simulink model "updated_target_driver_2026_withVariants_MPC"  (R2024b)
settings: Solver=FixedStepDiscrete  StartTime=0.0  StopTime=running_time  FixedStep=dt_s  RelTol=1e-3
values from neighbouring files (symbols this model uses):
  A = gamma_2*gamma_3*Thrust_desired    [force2voltage.m]
  a2_lb = -0.25    [target_driver_setup_2022_Ctrl_V_2_4.m]    (also in target_driver_setup_2022_Ctrl_V_2_4_geometric.m; target_driver_setup_mpc_12msdelay.m; target_driver_setup_mpc_andWLQP.m)
  a2_openloop = -0    (= 0)    [target_driver_setup_2022_Ctrl_V_2_4.m]    (also in target_driver_setup_2022_Ctrl_V_2_4_geometric.m; target_driver_setup_mpc_12msdelay.m; target_driver_setup_mpc_andWLQP.m)
  a2_ub = 0.25    [target_driver_setup_2022_Ctrl_V_2_4.m]    (also in target_driver_setup_2022_Ctrl_V_2_4_geometric.m; target_driver_setup_mpc_12msdelay.m; target_driver_setup_mpc_andWLQP.m)
  adaptive_flag = 0    [target_driver_setup_2022_Ctrl_V_2_4.m]    (also in target_driver_setup_2022_Ctrl_V_2_4_geometric.m; target_driver_setup_mpc_12msdelay.m = 1; target_driver_setup_mpc_andWLQP.m = 1)
  adaptive_gain = [gamma_adaptive, adaptive_roll_limit, adaptive_pitch_limit, adaptive_yaw_limit, c_2_adaptive, gamma_lateral_adaptive, adaptive_x_limit, adaptive_y_limit, adaptive_z_limit, c_1_adaptive]    [target_driver_setup_2022_Ctrl_V_2_4.m]    (also in target_driver_setup_2022_Ctrl_V_2_4_geometric.m; target_driver_setup_mpc_12msdelay.m; target_driver_setup_mpc_andWLQP.m)
  adaptive_lateral_flag = 0    [target_driver_setup_2022_Ctrl_V_2_4.m]    (also in target_driver_setup_2022_Ctrl_V_2_4_geometric.m; target_driver_setup_mpc_12msdelay.m = 1; target_driver_setup_mpc_andWLQP.m = 1)
  adaptive_pitch_init = 0    [target_driver_setup_2022_Ctrl_V_2_4.m]    (also in target_driver_setup_2022_Ctrl_V_2_4_geometric.m; target_driver_setup_mpc_12msdelay.m; target_driver_setup_mpc_andWLQP.m)
  adaptive_pitch_limit = 0.1/(scale^2)    (= 1e-07)    [target_driver_setup_2022_Ctrl_V_2_4.m]    (also in target_driver_setup_2022_Ctrl_V_2_4_geometric.m = 3e-07; target_driver_setup_mpc_12msdelay.m; target_driver_setup_mpc_andWLQP.m)
  adaptive_pitch_limit_low = -adaptive_pitch_limit    (= -1e-07)    [target_driver_setup_2022_Ctrl_V_2_4.m]    (also in target_driver_setup_2022_Ctrl_V_2_4_geometric.m = -3e-07; target_driver_setup_mpc_12msdelay.m; target_driver_setup_mpc_andWLQP.m)
  adaptive_roll_init = 0    [target_driver_setup_2022_Ctrl_V_2_4.m]    (also in target_driver_setup_2022_Ctrl_V_2_4_geometric.m; target_driver_setup_mpc_12msdelay.m; target_driver_setup_mpc_andWLQP.m)
  adaptive_roll_limit = 0.3/(scale^2)    (= 3e-07)    [target_driver_setup_2022_Ctrl_V_2_4.m]    (also in target_driver_setup_2022_Ctrl_V_2_4_geometric.m; target_driver_setup_mpc_12msdelay.m; target_driver_setup_mpc_andWLQP.m)
  adaptive_roll_limit_low = -adaptive_roll_limit    (= -3e-07)    [target_driver_setup_2022_Ctrl_V_2_4.m]    (also in target_driver_setup_2022_Ctrl_V_2_4_geometric.m; target_driver_setup_mpc_12msdelay.m; target_driver_setup_mpc_andWLQP.m)
  adaptive_x_init = 0    [target_driver_setup_2022_Ctrl_V_2_4.m]    (also in target_driver_setup_2022_Ctrl_V_2_4_geometric.m; target_driver_setup_mpc_12msdelay.m; target_driver_setup_mpc_andWLQP.m)
  adaptive_x_limit = 0.15/(scale)    (= 0.00015)    [target_driver_setup_2022_Ctrl_V_2_4.m]    (also in target_driver_setup_2022_Ctrl_V_2_4_geometric.m = 7.5e-05; target_driver_setup_mpc_12msdelay.m; target_driver_setup_mpc_andWLQP.m)
  adaptive_x_limit_low = -adaptive_x_limit    (= -0.00015)    [target_driver_setup_2022_Ctrl_V_2_4.m]    (also in target_driver_setup_2022_Ctrl_V_2_4_geometric.m = -7.5e-05; target_driver_setup_mpc_12msdelay.m; target_driver_setup_mpc_andWLQP.m)
  adaptive_y_init = 0    [target_driver_setup_2022_Ctrl_V_2_4.m]    (also in target_driver_setup_2022_Ctrl_V_2_4_geometric.m; target_driver_setup_mpc_12msdelay.m; target_driver_setup_mpc_andWLQP.m)
  adaptive_y_limit = 0.15/(scale)    (= 0.00015)    [target_driver_setup_2022_Ctrl_V_2_4.m]    (also in target_driver_setup_2022_Ctrl_V_2_4_geometric.m = 7.5e-05; target_driver_setup_mpc_12msdelay.m; target_driver_setup_mpc_andWLQP.m)
  adaptive_y_limit_low = -adaptive_y_limit    (= -0.00015)    [target_driver_setup_2022_Ctrl_V_2_4.m]    (also in target_driver_setup_2022_Ctrl_V_2_4_geometric.m = -7.5e-05; target_driver_setup_mpc_12msdelay.m; target_driver_setup_mpc_andWLQP.m)
  adaptive_yaw_init = 0    [target_driver_setup_2022_Ctrl_V_2_4.m]    (also in target_driver_setup_2022_Ctrl_V_2_4_geometric.m; target_driver_setup_mpc_12msdelay.m; target_driver_setup_mpc_andWLQP.m)
  adaptive_yaw_limit = 0.035/(scale^2)    (= 3.5e-08)    [target_driver_setup_2022_Ctrl_V_2_4.m]    (also in target_driver_setup_2022_Ctrl_V_2_4_geometric.m; target_driver_setup_mpc_12msdelay.m; target_driver_setup_mpc_andWLQP.m)
  adaptive_yaw_limit_low = -adaptive_yaw_limit    (= -3.5e-08)    [target_driver_setup_2022_Ctrl_V_2_4.m]    (also in target_driver_setup_2022_Ctrl_V_2_4_geometric.m; target_driver_setup_mpc_12msdelay.m; target_driver_setup_mpc_andWLQP.m)
  adaptive_z_init = 0/scale    (= 0)    [target_driver_setup_2022_Ctrl_V_2_4.m]    (also in target_driver_setup_2022_Ctrl_V_2_4_geometric.m; target_driver_setup_mpc_12msdelay.m; target_driver_setup_mpc_andWLQP.m)
  adaptive_z_limit = 0.20/(scale)    (= 0.0002)    [target_driver_setup_2022_Ctrl_V_2_4.m]    (also in target_driver_setup_2022_Ctrl_V_2_4_geometric.m = 0.0008; target_driver_setup_mpc_12msdelay.m = 0.0008; target_driver_setup_mpc_andWLQP.m = 0.0008)
  adaptive_z_limit_low = -adaptive_z_limit/1    (= -0.0002)    [target_driver_setup_2022_Ctrl_V_2_4.m]    (also in target_driver_setup_2022_Ctrl_V_2_4_geometric.m = -0.0008; target_driver_setup_mpc_12msdelay.m = -0.0008; target_driver_setup_mpc_andWLQP.m = -0.0008)
  att_s = 500    [target_driver_setup_2022_Ctrl_V_2_4.m]    (also in target_driver_setup_2022_Ctrl_V_2_4_geometric.m; target_driver_setup_mpc_12msdelay.m; target_driver_setup_mpc_andWLQP.m)
  b_1_d_desired = [1,0,0]    [target_driver_setup_2022_Ctrl_V_2_4.m]    (also in target_driver_setup_2022_Ctrl_V_2_4_geometric.m; target_driver_setup_mpc_12msdelay.m; target_driver_setup_mpc_andWLQP.m)
  closedloop_flag = 1    [target_driver_setup_2022_Ctrl_V_2_4.m]    (also in target_driver_setup_2022_Ctrl_V_2_4_geometric.m = 0; target_driver_setup_mpc_12msdelay.m = 0; target_driver_setup_mpc_andWLQP.m = 0)
  control_gain = [k_x,k_v, k_R, k_Omega, k_z, k_vz, k_Rx]    [target_driver_setup_2022_Ctrl_V_2_4.m]    (also in target_driver_setup_2022_Ctrl_V_2_4_geometric.m = [k_x,k_v,k_R,k_Omega_pitch,k_Omega_roll,k_z,k_vz,k_Rx]; target_driver_setup_mpc_12msdelay.m = [k_x, k_v, k_R, k_Omega, k_z, k_vz, k_Rx,                  k; target_driver_setup_mpc_andWLQP.m = [k_x, k_v, k_R, k_Omega, k_z, k_vz, k_Rx,                  k)
  delay = delay-vicon_sample_cycle/2    [target_driver_setup_2022_Ctrl_V_2_4.m]    (also in target_driver_setup_2022_Ctrl_V_2_4_geometric.m; target_driver_setup_mpc_12msdelay.m; target_driver_setup_mpc_andWLQP.m)
  drv_amp = abs((vleft_p2p-vright_p2p))/2+min(vleft_p2p,vright_p2p)    [Wing_traj_to_Voltage.m]    (also in force2voltage.m; target_driver_setup_2022_Ctrl_V_2_4.m = 300; target_driver_setup_2022_Ctrl_V_2_4_geometric.m = 133; target_driver_setup_mpc_12msdelay.m = 150)
  drv_bias = max_drv_bias    (= 300)    [target_driver_setup_2022_Ctrl_V_2_4.m]    (also in target_driver_setup_2022_Ctrl_V_2_4_geometric.m = 200; target_driver_setup_mpc_12msdelay.m = 200; target_driver_setup_mpc_andWLQP.m = 200)
  drv_pitch_left = vleft_pitch    [Wing_traj_to_Voltage.m]    (also in force2voltage.m = 0; target_driver_setup_2022_Ctrl_V_2_4.m = 0; target_driver_setup_2022_Ctrl_V_2_4_geometric.m = 0; target_driver_setup_mpc_12msdelay.m = 9.05)
  drv_pitch_right = vright_pitch    [Wing_traj_to_Voltage.m]    (also in force2voltage.m = 0; target_driver_setup_2022_Ctrl_V_2_4.m = 0; target_driver_setup_2022_Ctrl_V_2_4_geometric.m = 0; target_driver_setup_mpc_12msdelay.m = 9.05)
  drv_roll = (vleft_p2p-vright_p2p)/4    [Wing_traj_to_Voltage.m]    (also in force2voltage.m; target_driver_setup_2022_Ctrl_V_2_4.m = 0; target_driver_setup_2022_Ctrl_V_2_4_geometric.m = -0.001; target_driver_setup_mpc_12msdelay.m = -0.001)
  dt_s = 1e-3    (= 0.001)    [target_driver_setup_2022_Ctrl_V_2_4.m]    (also in target_driver_setup_2022_Ctrl_V_2_4_geometric.m = 0.0002; target_driver_setup_mpc_12msdelay.m = 0.0002; target_driver_setup_mpc_andWLQP.m = 0.0002)
  f_fin = f    (= 180)    [target_driver_setup_2022_Ctrl_V_2_4.m]    (also in target_driver_setup_2022_Ctrl_V_2_4_geometric.m = 155; target_driver_setup_mpc_12msdelay.m = 155; target_driver_setup_mpc_andWLQP.m = 155)
  f_int = f    (= 180)    [target_driver_setup_2022_Ctrl_V_2_4.m]    (also in target_driver_setup_2022_Ctrl_V_2_4_geometric.m = 155; target_driver_setup_mpc_12msdelay.m = 155; target_driver_setup_mpc_andWLQP.m = 155)
  g = 9.8    [target_driver_setup_2022_Ctrl_V_2_4.m]    (also in target_driver_setup_2022_Ctrl_V_2_4_geometric.m; target_driver_setup_mpc_12msdelay.m; target_driver_setup_mpc_andWLQP.m = 9.81; test_full_attitude_mpc.m = 9.81)
  I_moment_vec = [Ixx, Iyy, Izz]    [target_driver_setup_2022_Ctrl_V_2_4.m]    (also in target_driver_setup_2022_Ctrl_V_2_4_geometric.m; target_driver_setup_mpc_12msdelay.m; target_driver_setup_mpc_andWLQP.m)
  k_tau_vec = [k_tau_roll;k_tau_pitch]    [target_driver_setup_2022_Ctrl_V_2_4_geometric.m]    (also in target_driver_setup_mpc_12msdelay.m; target_driver_setup_mpc_andWLQP.m)
  landing_flag = 0    [target_driver_setup_2022_Ctrl_V_2_4.m]    (also in target_driver_setup_2022_Ctrl_V_2_4_geometric.m; target_driver_setup_mpc_12msdelay.m; target_driver_setup_mpc_andWLQP.m)
  landing_parameter = [start_delay+T,transition_rate, rising_time, falling_time, landing_rising_time, landing_z_decrease, landing_y_decrease, landing_x_decrease]    [target_driver_setup_2022_Ctrl_V_2_4.m]    (also in target_driver_setup_2022_Ctrl_V_2_4_geometric.m; target_driver_setup_mpc_12msdelay.m; target_driver_setup_mpc_andWLQP.m)
  low_bound = -8    [target_driver_setup_2022_Ctrl_V_2_4.m]    (also in target_driver_setup_2022_Ctrl_V_2_4_geometric.m = -5; target_driver_setup_mpc_12msdelay.m = -10; target_driver_setup_mpc_andWLQP.m = -10)
  low_bound_eR = -0.8    [target_driver_setup_2022_Ctrl_V_2_4.m]    (also in target_driver_setup_2022_Ctrl_V_2_4_geometric.m = -1.2; target_driver_setup_mpc_12msdelay.m = -1.2; target_driver_setup_mpc_andWLQP.m = -1.2)
  low_bound_vx = -0.5    [target_driver_setup_2022_Ctrl_V_2_4.m]    (also in target_driver_setup_2022_Ctrl_V_2_4_geometric.m; target_driver_setup_mpc_12msdelay.m; target_driver_setup_mpc_andWLQP.m)
  low_bound_vy = -0.5    [target_driver_setup_2022_Ctrl_V_2_4.m]    (also in target_driver_setup_2022_Ctrl_V_2_4_geometric.m; target_driver_setup_mpc_12msdelay.m; target_driver_setup_mpc_andWLQP.m)
  low_bound_vz = -0.5    [target_driver_setup_2022_Ctrl_V_2_4.m]    (also in target_driver_setup_2022_Ctrl_V_2_4_geometric.m; target_driver_setup_mpc_12msdelay.m; target_driver_setup_mpc_andWLQP.m)
  low_bound_x = -0.06    [target_driver_setup_2022_Ctrl_V_2_4.m]    (also in target_driver_setup_2022_Ctrl_V_2_4_geometric.m = -0.1; target_driver_setup_mpc_12msdelay.m = -0.6; target_driver_setup_mpc_andWLQP.m = -0.6)
  low_bound_y = -0.06    [target_driver_setup_2022_Ctrl_V_2_4.m]    (also in target_driver_setup_2022_Ctrl_V_2_4_geometric.m; target_driver_setup_mpc_12msdelay.m = -0.6; target_driver_setup_mpc_andWLQP.m = -0.6)
  low_bound_z = -0.04    [target_driver_setup_2022_Ctrl_V_2_4.m]    (also in target_driver_setup_2022_Ctrl_V_2_4_geometric.m; target_driver_setup_mpc_12msdelay.m = -0.1; target_driver_setup_mpc_andWLQP.m = -0.1)
  m = t <= t_zoom    [plot_roll_torque_cmd_vs_actual.m]    (also in plot_roll_torque_cmd_vs_actual_flightlog.m = t >= t0 & t <= t1; target_driver_setup_2022_Ctrl_V_2_4.m = 0.000124; target_driver_setup_2022_Ctrl_V_2_4_geometric.m = 8.5655e-05; target_driver_setup_mpc_12msdelay.m = 8.5655e-05)
  params_vec = [params_opt.delta_1, params_opt.delta_2, params_opt.delta_3,      params_opt.gamma_1, params_opt.gamma_2_1, params_opt.gamma_3,      params_opt.eta, params_opt.nu, params_opt.mu]'    [force2voltage_tuningSandbox.m]    (also in target_driver_setup_2022_Ctrl_V_2_4.m = [params_opt.delta_1, params_opt.delta_2, params_opt.delta_3,; target_driver_setup_2022_Ctrl_V_2_4_geometric.m = [params_opt.delta_1, params_opt.delta_2, params_opt.delta_3,; target_driver_setup_mpc_12msdelay.m = [params_opt.delta_1, params_opt.delta_2, params_opt.delta_3,; target_driver_setup_mpc_andWLQP.m = [params_opt.delta_1, params_opt.delta_2, params_opt.delta_3,)
  phase = 0    [target_driver_setup_2022_Ctrl_V_2_4.m]    (also in target_driver_setup_2022_Ctrl_V_2_4_geometric.m; target_driver_setup_mpc_12msdelay.m; target_driver_setup_mpc_andWLQP.m)
  r_desired = [default_x, default_y,z_desired]    [target_driver_setup_2022_Ctrl_V_2_4.m]    (also in target_driver_setup_2022_Ctrl_V_2_4_geometric.m; target_driver_setup_mpc_12msdelay.m; target_driver_setup_mpc_andWLQP.m)
  roll_offset_angle = 0    [target_driver_setup_2022_Ctrl_V_2_4.m]    (also in target_driver_setup_2022_Ctrl_V_2_4_geometric.m; target_driver_setup_mpc_12msdelay.m; target_driver_setup_mpc_andWLQP.m)
  running_time = start_delay+total_T    (= 9)    [target_driver_setup_2022_Ctrl_V_2_4.m]    (also in target_driver_setup_2022_Ctrl_V_2_4_geometric.m = 10; target_driver_setup_mpc_12msdelay.m = 0.5; target_driver_setup_mpc_andWLQP.m = 10)
  running_time_control = start_delay_control+total_T+0.0    (= 7.1)    [target_driver_setup_2022_Ctrl_V_2_4.m]    (also in target_driver_setup_2022_Ctrl_V_2_4_geometric.m = 10; target_driver_setup_mpc_12msdelay.m = 0.5; target_driver_setup_mpc_andWLQP.m = 10)
  sampling_f = 10000    [target_driver_setup_2022_Ctrl_V_2_4.m]    (also in target_driver_setup_2022_Ctrl_V_2_4_geometric.m = 5000; target_driver_setup_mpc_12msdelay.m = 5000; target_driver_setup_mpc_andWLQP.m = 5000)
  start_delay = 2.0    (= 2)    [target_driver_setup_2022_Ctrl_V_2_4.m]    (also in target_driver_setup_2022_Ctrl_V_2_4_geometric.m = 0; target_driver_setup_mpc_12msdelay.m = 0; target_driver_setup_mpc_andWLQP.m = 0)
  start_delay_control = start_delay + ramp_delay    (= 0.1)    [target_driver_setup_2022_Ctrl_V_2_4.m]    (also in target_driver_setup_2022_Ctrl_V_2_4_geometric.m = 0; target_driver_setup_mpc_12msdelay.m = 0; target_driver_setup_mpc_andWLQP.m = 0)
  T = 1    [target_driver_setup_2022_Ctrl_V_2_4.m]    (also in target_driver_setup_2022_Ctrl_V_2_4_geometric.m = 10; target_driver_setup_mpc_12msdelay.m = 0.5; target_driver_setup_mpc_andWLQP.m = 10; test_full_attitude_mpc.m = T0 + nu(1))
  task_flag = 0    [target_driver_setup_2022_Ctrl_V_2_4.m]    (also in target_driver_setup_2022_Ctrl_V_2_4_geometric.m; target_driver_setup_mpc_12msdelay.m; target_driver_setup_mpc_andWLQP.m)
  task_parameter = [radius_ref, frequency_ref, radius_ratio, lissajous_ratio, lissajous_delta, lissajous_amplitude_ratio,z_radius_ratio]    [target_driver_setup_2022_Ctrl_V_2_4.m]    (also in target_driver_setup_2022_Ctrl_V_2_4_geometric.m; target_driver_setup_mpc_12msdelay.m; target_driver_setup_mpc_andWLQP.m)
  upp_bound = 8    [target_driver_setup_2022_Ctrl_V_2_4.m]    (also in target_driver_setup_2022_Ctrl_V_2_4_geometric.m = 5; target_driver_setup_mpc_12msdelay.m = 10; target_driver_setup_mpc_andWLQP.m = 10)
  upp_bound_eR = 0.8    [target_driver_setup_2022_Ctrl_V_2_4.m]    (also in target_driver_setup_2022_Ctrl_V_2_4_geometric.m = 1.2; target_driver_setup_mpc_12msdelay.m = 1.2; target_driver_setup_mpc_andWLQP.m = 1.2)
  upp_bound_vx = 0.5    [target_driver_setup_2022_Ctrl_V_2_4.m]    (also in target_driver_setup_2022_Ctrl_V_2_4_geometric.m; target_driver_setup_mpc_12msdelay.m; target_driver_setup_mpc_andWLQP.m)
  upp_bound_vy = 0.5    [target_driver_setup_2022_Ctrl_V_2_4.m]    (also in target_driver_setup_2022_Ctrl_V_2_4_geometric.m; target_driver_setup_mpc_12msdelay.m; target_driver_setup_mpc_andWLQP.m)
  upp_bound_vz = 0.5    [target_driver_setup_2022_Ctrl_V_2_4.m]    (also in target_driver_setup_2022_Ctrl_V_2_4_geometric.m; target_driver_setup_mpc_12msdelay.m; target_driver_setup_mpc_andWLQP.m)
  upp_bound_x = 0.06    [target_driver_setup_2022_Ctrl_V_2_4.m]    (also in target_driver_setup_2022_Ctrl_V_2_4_geometric.m = 0.1; target_driver_setup_mpc_12msdelay.m = 0.6; target_driver_setup_mpc_andWLQP.m = 0.6)
  upp_bound_y = 0.06    [target_driver_setup_2022_Ctrl_V_2_4.m]    (also in target_driver_setup_2022_Ctrl_V_2_4_geometric.m; target_driver_setup_mpc_12msdelay.m = 0.6; target_driver_setup_mpc_andWLQP.m = 0.6)
  upp_bound_z = 0.04    [target_driver_setup_2022_Ctrl_V_2_4.m]    (also in target_driver_setup_2022_Ctrl_V_2_4_geometric.m; target_driver_setup_mpc_12msdelay.m = 0.1; target_driver_setup_mpc_andWLQP.m = 0.1)
  weights_vec = [ws; wds; wpr_xy;wpr_z; wpf; wvr_xy; wvr_z ... (first row only)    [target_driver_setup_2022_Ctrl_V_2_4_geometric.m]    (also in target_driver_setup_mpc_12msdelay.m; target_driver_setup_mpc_andWLQP.m)
undefined symbols (not defined in the file or in its folder): Com1, DiscIntNeverNeededParam, dspblkCoreblockFVToolHelper, gcbh, left_mapping, left_mapping_F_to_Phi, lp_den, lp_num, none, right_mapping, right_mapping_F_to_Phi, vlp_den, vlp_num
libraries: simulink x20, xpcseriallib x2, cstblocks x1, xpcnilib x1, xpcutilitieslib x1
(part 7 of 7)

== matlab function updated_target_driver_2026_withVariants_MPC/Geometric Controller/Geometric Controller ==
  data: thrust_desired output size=[1 1]; R_cur input; s_des input; omega input; roll_torque_desired output size=[1 1]; omega_desired input; omega_d_dot input; x_d_ddot input; e_x input; e_v input; e_R input; e_Omega input; control_gain input; I_moment_vec input; pitch_torque_desired output size=[1 1]; m input; g input; yaw_torque_desired output size=[1 1]; cntrl_enable input; adaptive_pitch input; adaptive_yaw input; adaptive_x input; adaptive_y input; adaptive_z input; weights_vec input; k_tau input
function [thrust_desired, roll_torque_desired, pitch_torque_desired, yaw_torque_desired] = upright_template_mpc(R_cur, s_des, omega, omega_desired, omega_d_dot, x_d_ddot, e_x, e_v, e_R, e_Omega, control_gain, I_moment_vec, m, g, cntrl_enable, adaptive_pitch, adaptive_yaw, adaptive_x, adaptive_y, adaptive_z, weights_vec, k_tau)
% vofunction [thrust_desired, roll_torque_desired, pitch_torque_desired, yaw_torque_desired] = ...
%     upright_template_mpc(R_cur,s_des, omega, omega_desired, omega_d_dot, ...
%     x_d_ddot,e_x,e_v,e_R,e_Omega,control_gain,I_moment_vec, m, g, cntrl_enable, ...
%     adaptive_pitch, adaptive_yaw, adaptive_x,adaptive_y, adaptive_z,weights_vec, ...
%     k_tau)
%#codegen
% Monolithic "upright MPC" (template controller), after Chen et al.
% robobee3d/template/template_controllers.py :: UprightMPC2, augmented with
% a first-order torque-actuation lag model measured on THIS plant
% (system-id: pitch moment develops with ~6 ms dead time + ~6-15 ms lag;
% approximated here as a single 12 ms first-order lag on both moment axes).
%
% One QP, solved every controller step, directly outputs thrust and
% roll/pitch torques from the current state and the references
% (desired position via e_x/e_v, desired body-z vector via the s_des
% input). No attitude cascade, no heading (b_1_d) reference. Yaw is NOT
% controlled: yaw torque = 0.
%
% Template model (reduced attitude, yaw-free):
%   y  = [p; s],   s  = R*e3   (body z-axis in world frame)
%   dy = [v; ds],  ds = -R*e3hat*omega_body
%   v_dot  = T*s - g*e3  ~ T0*s + s0*utilde - g*e3   (bilinear, linearized
%                                                     about persistent T0
%                                                     and current s0)
%   ds_dot = Btau*[tauX_applied; tauY_applied]
%   tau_applied_dot = (tau_cmd - tau_applied)/tau_lag   (actuation lag)
%   u = [utilde; tauX_cmd; tauY_cmd]
%
% The QP is condensed to a dense box-constrained problem in U (nu*N vars)
% and solved with the same deterministic coordinate-descent used by the
% previous controllers (OSQP is not available under codegen here).
%
% Internally everything runs in the template's units (mm, ms, mg):
%   force:  1 mg*mm/ms^2  = 1e-3 N
%   torque: 1 mg*mm^2/ms^2 = 1e-6 N*m
%
% Unused inputs (kept for block signature compatibility): omega_desired,
% omega_d_dot, e_R, e_Omega, control_gain, adaptive_*.

% -------------------------------------------------------------------------
% Fixed dimensions for Simulink codegen
% -------------------------------------------------------------------------
R_cur = reshape(R_cur, 9, 1);
s_des = reshape(s_des, 3, 1);
omega = reshape(omega, 3, 1);
omega_desired = reshape(omega_desired, 3, 1);     %#ok<NASGU>
omega_d_dot = reshape(omega_d_dot, 3, 1);         %#ok<NASGU>
x_d_ddot = reshape(x_d_ddot, 3, 1);
e_x = reshape(e_x, 3, 1);
e_v = reshape(e_v, 3, 1);
e_R = reshape(e_R, 3, 1);                         %#ok<NASGU>
e_Omega = reshape(e_Omega, 3, 1);                 %#ok<NASGU>
control_gain = reshape(control_gain, 10, 1);      %#ok<NASGU>
I_moment_vec = reshape(I_moment_vec, 3, 1);
weights_vec = reshape(weights_vec, 14, 1);
k_tau = reshape(k_tau, 2, 1);
m = m(1);
g = g(1);
cntrl_enable = cntrl_enable(1);
adaptive_pitch = adaptive_pitch(1);               %#ok<NASGU>
adaptive_yaw = adaptive_yaw(1);                   %#ok<NASGU>
adaptive_x = adaptive_x(1);                       %#ok<NASGU>
adaptive_y = adaptive_y(1);                       %#ok<NASGU>
adaptive_z = adaptive_z(1);                       %#ok<NASGU>

% -------------------------------------------------------------------------
% MPC constants (template units: mm, ms, mg)
% -------------------------------------------------------------------------
N = 8;          % horizon steps (template default 3; 8 -> 40 ms preview,
                % enough to see through the 12 ms actuation lag)
dt = 6.45;       % [ms] prediction step (template default). 
ny = 6;
nu = 3;
nx = 2*ny + 2;  % [y_err; dy_err; tauX_applied; tauY_applied]
nU = nu*N;

controller_dt = 0.2;   % [ms] Simulink sample time of this block (2e-4 s)
% tau_lag = (1/155)*1e3*0.1;        % [ms] moment actuation lag (system-id: dead+lag)
% tau_lag = 12; 
% tau_lag = 12.9 / (-log(0.05));  % = 4.306 ms
tau_lag = 10; 

% Template-derived weights, retuned for THIS plant (probe-based scan
% matched to the takeoff-transient torque levels the proven geometric/
% delay-MPC controller used: ~1 uNm at 10-20 deg tilt wobble). With the
% vehicle's huge torque authority (15 uNm ~ 7400 rad/s^2) and the ~18 ms
% effective moment actuation delay, the template's wmom=1e-2 makes torque
% free and commands bang-bang between the rails (flips the bee at
% takeoff); stiff variants (wmom=1) still oscillated through the delay.
% These values give ~0.7 uNm per 0.2 rad tilt, ~0.4 uNm per 5 rad/s rate,
% ~0.15 uNm per 2 cm/s lateral velocity error.
% ws      = 3.0e1;    % running orientation-vector weight
% wds     = 1.5e2;    % running orientation-rate weight
% wpr     = 1.0;      % running position weight
% wpf     = 5.0;      % final position weight
% wvr     = 1.0e3;    % running velocity weight
% wvf     = 2.0e3;    % final velocity weight
% wthrust = 1.0e-1;   % specific-thrust-correction effort
% wmom    = 3.0e0;    % torque effort

ws      = weights_vec(1);   % running orientation-vector weight
wds     = weights_vec(2);   % running orientation-rate weight
wpr_xy  = weights_vec(3);   % running position weight
wpr_z   = weights_vec(4);
wpf     = weights_vec(5);   % final position weight
wvr_xy  = weights_vec(6);   % running horizontal-velocity weight
wvr_z   = weights_vec(7);   % running vertical-velocity weight
wvf_xy  = weights_vec(8);   % final horizontal-velocity weight
wvf_z   = weights_vec(9);   % final vertical-velocity weight
wthrust     = weights_vec(10); % specific-thrust-correction effort
wmom        = weights_vec(11); % roll/pitch torque magnitude effort
wdmom_roll  = weights_vec(12); % roll torque-change penalty
wdmom_pitch = weights_vec(13); % pitch torque-change penalty
wdthrust    = weights_vec(14); % commanded specific-thrust-change penalty


% Actuator limits (SI, same as previous controllers)
thrust_min_N = 0.8e-3;   % [N]
thrust_max_N = 1.6e-3;   % [N]
roll_max_Nm  = 15e-6;   %  [N*m]
pitch_max_Nm = 10.0e-6;   % [N*m]

% -------------------------------------------------------------------------
% Unit conversion to template units
% -------------------------------------------------------------------------
m_t = m * 1.0e6;                 % kg      -> mg
g_t = g * 1.0e-3;                % m/s^2   -> mm/ms^2
ex_t = e_x * 1.0e3;              % m       -> mm
ev_t = e_v;                      % m/s == mm/ms
om_t = omega * 1.0e-3;           % rad/s   -> rad/ms
xdd_t = x_d_ddot * 1.0e-3;       % m/s^2   -> mm/ms^2
Ib_t = I_moment_vec * 1.0e12;    % kg*m^2  -> mg*mm^2

Tmin_sp = thrust_min_N * 1.0e3 / max(m_t, 1.0e-9);  % specific thrust [mm/ms^2]
Tmax_sp = thrust_max_N * 1.0e3 / max(m_t, 1.0e-9);
tau_roll_max  = roll_max_Nm  * 1.0e6;   % N*m -> mg*mm^2/ms^2
tau_pitch_max = pitch_max_Nm * 1.0e6;

% -------------------------------------------------------------------------
% Persistent controller state: thrust linearization point T0 and the
% estimated APPLIED moments (hidden actuator states behind the lag)
% -------------------------------------------------------------------------
persistent T0 tau_applied thrust_cmd_prev_sp tau_cmd_prev U_prev
if isempty(T0)
    T0 = 0.0;
end
if isempty(tau_applied)
    tau_applied = zeros(2,1);
end
if isempty(thrust_cmd_prev_sp)
    thrust_cmd_prev_sp = 0.0;
end
if isempty(tau_cmd_prev)
    tau_cmd_prev = zeros(2,1);
end
if isempty(U_prev)
    U_prev = zeros(nU,1);
end

% -------------------------------------------------------------------------
% Soft-start envelope: cntrl_enable is the model's engagement ramp (the
% Cntrl_enable saturating ramp in Open_Closed_loop_selection, 0 -> 1).
% Rather than rate-limiting outputs externally (which the QP could not see
% and would fight), the ramp scales the QP's own constraint boxes: the
% thrust ceiling follows the ramp from zero and the torque boxes open from
% 30% to 100%. While disabled the controller state is held at rest so
% engagement starts bumplessly.
% -------------------------------------------------------------------------
en = cntrl_enable;
if en < 0.0
    en = 0.0;
elseif en > 1.0
    en = 1.0;
end
if en < 0.01
    T0 = 0.0;
    tau_applied = zeros(2,1);
    thrust_cmd_prev_sp = 0.0;
    tau_cmd_prev = zeros(2,1);
    U_prev = zeros(nU,1);
end
T_ceiling = en * Tmax_sp;                      % thrust ceiling rides the ramp
T_floor   = min(Tmin_sp, T_ceiling);           % floor engages once ceiling passes it
tau_roll_eff  = (0.3 + 0.7*en) * tau_roll_max; % torque boxes open 30% -> 100%
tau_pitch_eff = (0.3 + 0.7*en) * tau_pitch_max;

% -------------------------------------------------------------------------
% Current reduced-attitude state
% -------------------------------------------------------------------------
Rot = [R_cur(1), R_cur(2), R_cur(3); ...
       R_cur(4), R_cur(5), R_cur(6); ...
       R_cur(7), R_cur(8), R_cur(9)];

s0 = [R_cur(3); R_cur(6); R_cur(9)];          % R*e3, third column
sdes = s_des / max(norm(s_des), 1.0e-9);      % desired body-z, normalized

e3h = [0, -1, 0; 1, 0, 0; 0, 0, 0];           % hat([0;0;1])
Ibi = [1/max(Ib_t(1),1e-9), 0, 0; 0, 1/max(Ib_t(2),1e-9), 0; 0, 0, 1/max(Ib_t(3),1e-9)];

k_tau_roll = k_tau(1); 
k_tau_pitch = k_tau(2); 
BtauFull = -Rot * e3h * Ibi;
Btau = BtauFull(:, 1:2) * diag([k_tau_roll, k_tau_pitch]);                      % no yaw torque column

ds0 = -Rot * e3h * om_t;                      % s-rate from body omega

% Error state x0 = [e_p; e_s; e_v; e_ds; tau_applied], refs: sdes, ds_des=0
es0 = s0 - sdes;
x0 = [ex_t; es0; ev_t; ds0; tau_applied];

% Affine drift in error coordinates:
% e_v_dot = T0*e_s + s0*utilde + (T0*sdes - g*e3 - xdd_des)
d_v = T0*sdes - [0;0;g_t] - xdd_t;

% -------------------------------------------------------------------------
% Discrete error dynamics  x_{k+1} = Ad*x_k + Bd*u_k + cd
% indices: e_p 1:3, e_s 4:6, e_v 7:9, e_ds 10:12, tau_applied 13:14
% -------------------------------------------------------------------------
beta = 1.0 - exp(-dt / tau_lag);          % first-order lag step fraction (Euler)
if beta > 1.0
    beta = 1.0;
end

% Per-axis rotational damping from open-loop step ID (b in 1/s):
%   roll  (omega_x):  b_roll  = +47   real wing counter-torque (stable)
%   pitch (omega_y):  b_pitch = -30   ANTI-damped -> unstable open-loop mode
% Reduced-attitude swap (ds = -R*e3hat*omega): ds_x = omega_y (pitch) -> row 10,
% ds_y = -omega_x (roll) -> row 11. So pitch damping goes on Ad(10,10).
b_roll  =  47.0;
b_pitch = -30.0;
decay_pitch = 1.0 - b_pitch * (dt*1.0e-3);   % ds_x / state 10  (= 1.19, >1)
decay_roll  = 1.0 - b_roll  * (dt*1.0e-3);   % ds_y / state 11  (= 0.70)
% CRITICAL: do NOT clamp the pitch value down to 1. The pitch mode really
% grows, and the MPC must predict that to command torque early enough.
decay_pitch = min(max(decay_pitch, 0.0), 1.5);   % allow >1, cap for safety
decay_roll  = min(max(decay_roll,  0.0), 1.5);


Ad = eye(nx);
for i = 1:3
    Ad(i, 6+i) = dt;                           % e_p += dt*e_v
    Ad(3+i, 9+i) = dt;                         % e_s += dt*e_ds
    Ad(6+i, 3+i) = dt*T0;                      % e_v += dt*T0*e_s
end
% e_ds += dt*Btau*tau_applied  (moments act through the lag state)

% Ad(10,10) = rot_decay; 
% Ad(11,11) = rot_decay; 
% Ad(12,12) = rot_decay; 
Ad(10,10) = decay_pitch;
Ad(11,11) = decay_roll;
Ad(12,12) = 1.0;          % ds_z ~ 0 at hover; no ID data, leave undamped

Ad(10, 13) = dt*Btau(1,1);  Ad(10, 14) = dt*Btau(1,2);
Ad(11, 13) = dt*Btau(2,1);  Ad(11, 14) = dt*Btau(2,2);
Ad(12, 13) = dt*Btau(3,1);  Ad(12, 14) = dt*Btau(3,2);
% tau_applied += beta*(tau_cmd - tau_applied)
Ad(13, 13) = 1.0 - beta;
Ad(14, 14) = 1.0 - beta;

Bd = zeros(nx, nu);
Bd(7, 1) = dt*s0(1);                           % thrust correction -> e_v
Bd(8, 1) = dt*s0(2);
Bd(9, 1) = dt*s0(3);
Bd(13, 2) = beta;                              % tau commands -> lag states
Bd(14, 3) = beta;

cd = zeros(nx,1);
cd(7) = dt*d_v(1);
cd(8) = dt*d_v(2);
cd(9) = dt*d_v(3);

% -------------------------------------------------------------------------
% Stage weights: x = [e_p(3); e_s(3); e_v(3); e_ds(3); tau_app(2)]
% -------------------------------------------------------------------------
Qrun = [wpr_xy; wpr_xy; wpr_z; ...
        ws; ws; ws; ...
        wvr_xy; wvr_xy; wvr_z; ...
        wds; wds; wds; ...
        0; 0];

Qfin = [wpf; wpf; wpf; ...
        ws; ws; ws; ...
        wvf_xy; wvf_xy; wvf_z; ...
        wds; wds; wds; ...
        0; 0];
Rdiag = [wthrust; wmom; wmom];

% -------------------------------------------------------------------------
% Condense:  x_k = Phi_k*x0 + sum_j G(k,j)*u_j + w_k,  k = 1..N
% H = sum_k G_k' Q_k G_k + Rbar,  h = sum_k G_k' Q_k (Phi_k x0 + w_k)
% -------------------------------------------------------------------------
Gamma = zeros(nx*N, nU);
xfree = zeros(nx*N, 1);

for k = 1:N
    % free response (with affine drift)
    if k == 1
        xfree((k-1)*nx+1:k*nx) = Ad*x0 + cd;
    else
        xfree((k-1)*nx+1:k*nx) = Ad*xfree((k-2)*nx+1:(k-1)*nx) + cd;
    end
    % input response blocks: G(k,j) = Ad^(k-j-1)*Bd for j = 0..k-1
    for j = 1:k
        if j == k
            Gblk = Bd;
        else
            Gprev = Gamma((k-2)*nx+1:(k-1)*nx, (j-1)*nu+1:j*nu);
            Gblk = Ad*Gprev;
        end
        Gamma((k-1)*nx+1:k*nx, (j-1)*nu+1:j*nu) = Gblk;
    end
end

H = zeros(nU, nU);
h = zeros(nU, 1);
for k = 1:N
    if k == N
        Qk = Qfin;
    else
        Qk = Qrun;
    end
    Gk = Gamma((k-1)*nx+1:k*nx, :);
    xf = xfree((k-1)*nx+1:k*nx);
    GkQ = Gk' .* repmat(Qk', nU, 1);       % Gk' * diag(Qk)
    H = H + GkQ * Gk;
    h = h + GkQ * xf;
end
for k = 1:N
    base = (k-1)*nu;
    H(base+1, base+1) = H(base+1, base+1) + Rdiag(1);
    H(base+2, base+2) = H(base+2, base+2) + Rdiag(2);
    H(base+3, base+3) = H(base+3, base+3) + Rdiag(3);
end

% -------------------------------------------------------------------------
% Input-change penalties:
%   0.5*wdthrust*(T_cmd,0 - T_cmd,prev)^2
% + 0.5*wdmom_roll *(tau_x,0 - tau_x,prev)^2
% + 0.5*wdmom_pitch*(tau_y,0 - tau_y,prev)^2
% + sum 0.5*w*(u_k - u_k-1)^2 over the horizon.
%
% Each predicted absolute specific-thrust command is T0 + utilde_k.
% Since T0 is constant within one condensed QP, successive absolute-thrust
% differences equal successive utilde differences. For the first move,
% compare utilde_0 with thrust_cmd_prev_sp - T0 so that the penalty remains
% correct even if T0 and the previously issued thrust ever differ.
% QP convention: min 0.5*U'*H*U + h'*U.
% -------------------------------------------------------------------------
utilde_prev_ref = thrust_cmd_prev_sp - T0;
for k = 1:N
    idx_thrust = (k-1)*nu + 1;
    idx_roll  = (k-1)*nu + 2;
    idx_pitch = (k-1)*nu + 3;

    if k == 1
        H(idx_thrust,idx_thrust) = ...
            H(idx_thrust,idx_thrust) + wdthrust;
        h(idx_thrust) = h(idx_thrust) - wdthrust*utilde_prev_ref;

        H(idx_roll,idx_roll) = H(idx_roll,idx_roll) + wdmom_roll;
        h(idx_roll) = h(idx_roll) - wdmom_roll*tau_cmd_prev(1);

        H(idx_pitch,idx_pitch) = H(idx_pitch,idx_pitch) + wdmom_pitch;
        h(idx_pitch) = h(idx_pitch) - wdmom_pitch*tau_cmd_prev(2);
    else
        idx_thrust_prev = idx_thrust - nu;
        idx_roll_prev  = idx_roll  - nu;
        idx_pitch_prev = idx_pitch - nu;

        H(idx_thrust,idx_thrust) = ...
            H(idx_thrust,idx_thrust) + wdthrust;
        H(idx_thrust_prev,idx_thrust_prev) = ...
            H(idx_thrust_prev,idx_thrust_prev) + wdthrust;
        H(idx_thrust,idx_thrust_prev) = ...
            H(idx_thrust,idx_thrust_prev) - wdthrust;
        H(idx_thrust_prev,idx_thrust) = ...
            H(idx_thrust_prev,idx_thrust) - wdthrust;

        H(idx_roll,idx_roll) = H(idx_roll,idx_roll) + wdmom_roll;
        H(idx_roll_prev,idx_roll_prev) = ...
            H(idx_roll_prev,idx_roll_prev) + wdmom_roll;
        H(idx_roll,idx_roll_prev) = H(idx_roll,idx_roll_prev) - wdmom_roll;
        H(idx_roll_prev,idx_roll) = H(idx_roll_prev,idx_roll) - wdmom_roll;

        H(idx_pitch,idx_pitch) = H(idx_pitch,idx_pitch) + wdmom_pitch;
        H(idx_pitch_prev,idx_pitch_prev) = ...
            H(idx_pitch_prev,idx_pitch_prev) + wdmom_pitch;
        H(idx_pitch,idx_pitch_prev) = H(idx_pitch,idx_pitch_prev) - wdmom_pitch;
        H(idx_pitch_prev,idx_pitch) = H(idx_pitch_prev,idx_pitch) - wdmom_pitch;
    end
end

% -------------------------------------------------------------------------
% Box constraints per stage: thrust lims on utilde, actuator lims on torques
% -------------------------------------------------------------------------
Umin = zeros(nU,1);
Umax = zeros(nU,1);
for k = 1:N
    base = (k-1)*nu;
    Umin(base+1) = T_floor - T0;
    Umax(base+1) = T_ceiling - T0;
    Umin(base+2) = -tau_roll_eff;
    Umax(base+2) =  tau_roll_eff;
    Umin(base+3) = -tau_pitch_eff;
    Umax(base+3) =  tau_pitch_eff;
end

% -------------------------------------------------------------------------
% Receding-horizon warm start
%
% Previous solution:
%   U_prev = [u_0; u_1; ...; u_(N-1)]
%
% Initial guess for the new QP:
%   U_init = [u_1; u_2; ...; u_(N-1); u_(N-1)]
%
% This warm-starts the decision vector used by coordinate descent. The
% gradient is still recomputed from the current H, h, and current iterate.
% -------------------------------------------------------------------------
% U_init = zeros(nU,1);
% for k = 1:N-1
%     dst_base = (k-1)*nu;
%     src_base = k*nu;
% 
%     U_init(dst_base+1) = U_prev(src_base+1);
%     U_init(dst_base+2) = U_prev(src_base+2);
%     U_init(dst_base+3) = U_prev(src_base+3);
% end
% 
% % Repeat the previous terminal input at the end of the shifted sequence.
% last_base = (N-1)*nu;
% U_init(last_base+1) = U_prev(last_base+1);
% U_init(last_base+2) = U_prev(last_base+2);
% U_init(last_base+3) = U_prev(last_base+3);

U_init = U_prev; 

U = solve_box_qp_coordinate_descent( ...
    H, h, Umin, Umax, nU, U_init);

% Save the optimized horizon for the next MPC update.
U_prev = U;

% -------------------------------------------------------------------------
% Apply first input; advance linearization point (template: T0 += utilde0)
% and propagate the applied-moment estimate at the CONTROLLER rate
% -------------------------------------------------------------------------
utilde0 = U(1);
tau_x_t = U(2);
tau_y_t = U(3);

T0 = T0 + utilde0 * controller_dt/dt;
if T0 < T_floor
    T0 = T_floor;
elseif T0 > T_ceiling
    T0 = T_ceiling;
end
thrust_cmd_prev_sp = T0;

beta_c = 1.0 - exp(-controller_dt / tau_lag);
tau_applied(1) = tau_applied(1) + beta_c*(tau_x_t - tau_applied(1));
tau_applied(2) = tau_applied(2) + beta_c*(tau_y_t - tau_applied(2));

tau_cmd_prev(1) = tau_x_t;
tau_cmd_prev(2) = tau_y_t;

% Convert back to SI
thrust_desired = m_t * T0 * 1.0e-3;            % mg*mm/ms^2 -> N
roll_torque_desired  = tau_x_t * 1.0e-6;       % mg*mm^2/ms^2 -> N*m
pitch_torque_desired = tau_y_t * 1.0e-6;
yaw_torque_desired   = 0.0;                    % yaw not controlled

% Final SI saturations (redundant with QP boxes; cheap insurance)
thrust_desired = clamp_scalar(thrust_desired, 0.0, thrust_max_N);
roll_torque_desired = clamp_scalar(roll_torque_desired, -roll_max_Nm, roll_max_Nm);
pitch_torque_desired = clamp_scalar(pitch_torque_desired, -pitch_max_Nm, pitch_max_Nm);

end

function y = clamp_scalar(x, xmin, xmax)
%#codegen
y = x;
if y > xmax
    y = xmax;
elseif y < xmin
    y = xmin;
end
end

function U = solve_box_qp_coordinate_descent( ...
    H, h, Umin, Umax, nU, U_init)
%#codegen
% min 0.5*U'*H*U + h'*U  s.t. Umin <= U <= Umax
%
% Warm-start from the shifted solution of the previous MPC update.
U = reshape(U_init, nU, 1);

% Project the warm start into the current feasible box because the bounds
% can change with the engagement ramp and thrust linearization point.
for i = 1:nU
    if U(i) < Umin(i)
        U(i) = Umin(i);
    elseif U(i) > Umax(i)
        U(i) = Umax(i);
    end
end
% Fixed iteration count keeps generated code deterministic.
for iter = 1:20
    for i = 1:nU
        grad_i = h(i);
        for j = 1:nU
            grad_i = grad_i + H(i,j) * U(j);
        end
        U(i) = U(i) - grad_i / max(H(i,i), 1.0e-18);
        if U(i) < Umin(i)
            U(i) = Umin(i);
        elseif U(i) > Umax(i)
            U(i) = Umax(i);
        end
    end
end
end

== matlab function updated_target_driver_2026_withVariants_MPC/Open_Closed_loop_selection/MATLAB Function4 ==
  data: openloop_control input; closedloop_control input; drv_amp_final output; closedloop_flag input; drv_pch_final_left output; drv_pch_final_right output; drv_roll_final output; a2_final output
function [drv_amp_final, drv_pch_final_left,drv_pch_final_right, drv_roll_final, a2_final] = fcn(openloop_control, closedloop_control, closedloop_flag)

if closedloop_flag==1
    drv_amp_final =closedloop_control(1);
    drv_pch_final_left =closedloop_control(2);
		drv_pch_final_right =closedloop_control(3);
    drv_roll_final=closedloop_control(4);
		a2_final=closedloop_control(5);
else
    drv_amp_final =openloop_control(1);
    drv_pch_final_left =openloop_control(2);
		drv_pch_final_right =openloop_control(3);
    drv_roll_final=openloop_control(4);
		a2_final=openloop_control(5);
		
end

== matlab function updated_target_driver_2026_withVariants_MPC/Variant Subsystem/Simulation/MATLAB Function ==
  data: time output; dt_s input; left_voltage_v input; right_voltage_v input; bias_voltage_v input; x output; y output; z output; alpha_rad output; beta_rad output; gamma_rad output
function [time,x,y,z,alpha_rad,beta_rad,gamma_rad] = fcn(dt_s, left_voltage_v, right_voltage_v, bias_voltage_v)
%#codegen

pose = robobee_tcp_step_codegen(dt_s, left_voltage_v, right_voltage_v, bias_voltage_v);

time      = pose(1);
x         = pose(2);
y         = pose(3);
z         = pose(4);
alpha_rad = pose(5);
beta_rad  = pose(6);
gamma_rad = pose(7);

end
